simulink model "TwoLinkRobotOL"  (R2016b)
settings: Solver=VariableStepAuto  StartTime=0.0  StopTime=5  RelTol=1e-5
values from neighbouring files (symbols this model uses):
  alpha = RobotParam.alpha    [twoLinkInverseKinematics.m]    (also in twoLinkRobot_BuildLTVModel.m = 0.4425)
  beta = RobotParam.beta    [twoLinkInverseKinematics.m]    (also in twoLinkRobot_BuildLTVModel.m = 0.09)
  delta = RobotParam.delta    [twoLinkInverseKinematics.m]    (also in twoLinkRobot_BuildLTVModel.m = 0.105)
  eta0 = evalt(etabar,T0)    [twoLinkRobot_BuildLTVModel.m]
undefined symbols (not defined in the file): d, taubar
settings Model: Creator=pjseiler  LastModifiedBy=pjseiler

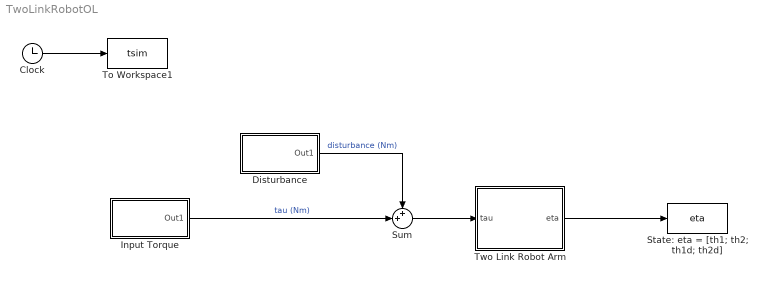
== system TwoLinkRobotOL ==
  Clock : Clock
  Disturbance : Subsystem  mask(Time-Varying Matrix){M=d, vec1D=on}
      mask prompts: M "Time-Varying Matrix"; vec1D "Interpret vector parameters as 1-D"
      mask help: Output the value of the specified time-varying matrix evaluated at the current simulation time. If the 'Time-Varying Matrix' parameter is M then the output at simulation time t is given by evalt(M,t). If M is a vector and the 'Interpret vector parameters as 1-D' is on, then the output is treated as a 1-D array. Otherwise the output is a matrix with the same dimensions as M.
      mask init:
      | if isequal(M.InterpolationMethod,'Spline') && ...
      |         isempty(M.SplineData)
      |     M = getSplineData(M);
      | end
      | fh = @(t) evalt(M,t);
      | szM = size(M);
      | if vec1D==1 && ndims(M)==2 && any(szM==1)
      |     dim = max(szM);
      | else
      |     dim = szM;
      | end
  Input Torque : Subsystem  mask(Time-Varying Matrix){M=taubar, vec1D=on}
      mask prompts: M "Time-Varying Matrix"; vec1D "Interpret vector parameters as 1-D"
      mask help: Output the value of the specified time-varying matrix evaluated at the current simulation time. If the 'Time-Varying Matrix' parameter is M then the output at simulation time t is given by evalt(M,t). If M is a vector and the 'Interpret vector parameters as 1-D' is on, then the output is treated as a 1-D array. Otherwise the output is a matrix with the same dimensions as M.
      mask init: same as TwoLinkRobotOL/Disturbance
  State: eta = [th1; th2; th1d; th2d] : ToWorkspace  VariableName=eta  SampleTime=-1
  Sum : Sum  Inputs=++|
  To Workspace1 : ToWorkspace  VariableName=tsim  SampleTime=-1
  Two Link Robot Arm : Subsystem
  wires:
  Disturbance/1(Out1) -> Sum/1  "disturbance (Nm)"
  Input Torque/1(Out1) -> Sum/2  "tau (Nm)"
  Clock/1 -> To Workspace1/1
  Sum/1 -> Two Link Robot Arm/1(tau)
  Two Link Robot Arm/1(eta) -> State: eta = [th1; th2; th1d; th2d]/1

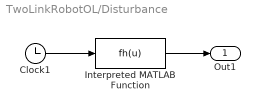
== system TwoLinkRobotOL/Disturbance ==
  Clock1 : Clock
  Interpreted MATLAB Function : MATLABFcn  MATLABFcn=fh(u)  OutputDimensions=dim  Output1D=off
  Out1 : Outport
  wires:
  Clock1/1 -> Interpreted MATLAB Function/1
  Interpreted MATLAB Function/1 -> Out1/1

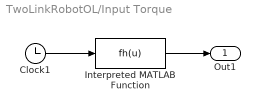
== system TwoLinkRobotOL/Input Torque ==
  Clock1 : Clock
  Interpreted MATLAB Function : MATLABFcn  MATLABFcn=fh(u)  OutputDimensions=dim  Output1D=off
  Out1 : Outport
  wires:
  Interpreted MATLAB Function/1 -> Out1/1
  Clock1/1 -> Interpreted MATLAB Function/1

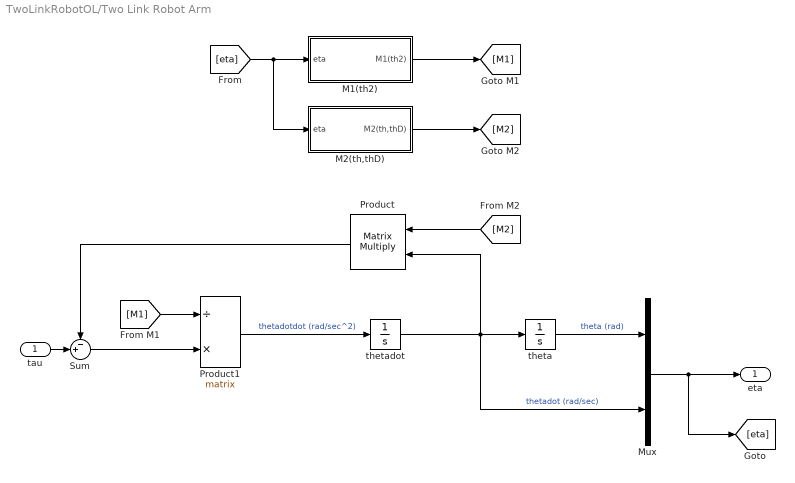
== system TwoLinkRobotOL/Two Link Robot Arm ==
  tau : Inport
  M1(th2) : Subsystem  TreatAsAtomicUnit=on
  M2(th,thD) : Subsystem  TreatAsAtomicUnit=on
  Mux : Mux  Inputs=2
  Product : Product  Inputs=**  Multiplication=Matrix(*)
  Product1 : Product  Inputs=/*  Multiplication=Matrix(*)
  Sum : Sum  Inputs=-+|
  theta : Integrator  InitialCondition=eta0(1:2)
  thetadot : Integrator  InitialCondition=eta0(3:4)
  eta : Outport
  wires:
  thetadot/1 -> Mux/2, Product/2, theta/1  "thetadot (rad/sec)"
  Sum/1 -> Product1/2
  Product/1 -> Sum/1
  [M1] -> Product1/1
  Product1/1 -> thetadot/1  "thetadotdot (rad/sec^2)"
  theta/1 -> Mux/1  "theta (rad)"
  M1(th2)/1(M1(th2)) -> [M1]
  [M2] -> Product/1
  M2(th,thD)/1(M2(th,thD)) -> [M2]
  [eta] -> M2(th,thD)/1(eta), M1(th2)/1(eta)
  Mux/1 -> [eta], eta/1
  tau/1 -> Sum/2

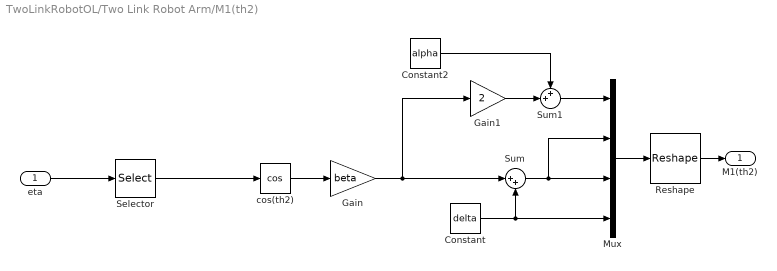
== system TwoLinkRobotOL/Two Link Robot Arm/M1(th2) ==
  eta : Inport
  Constant : Constant  Value=delta
  Constant2 : Constant  Value=alpha
  Gain : Gain  Gain=beta
  Gain1 : Gain  Gain=2
  Mux : Mux
  Reshape : Reshape  OutputDimensionality=Customize  OutputDimensions=[2 2]
  Selector : Selector  InputPortWidth=4  IndexOptions=Index vector (dialog)  Indices=2  OutputSizes=1
  Sum : Sum  Inputs=|++
  Sum1 : Sum  Inputs=++|
  cos(th2) : Trigonometry  Operator=cos
  M1(th2) : Outport
  wires:
  Reshape/1 -> M1(th2)/1
  Mux/1 -> Reshape/1
  Constant/1 -> Mux/4, Sum/2
  Sum/1 -> Mux/3, Mux/2
  cos(th2)/1 -> Gain/1
  Gain/1 -> Gain1/1, Sum/1
  Constant2/1 -> Sum1/1
  Sum1/1 -> Mux/1
  Gain1/1 -> Sum1/2
  eta/1 -> Selector/1
  Selector/1 -> cos(th2)/1

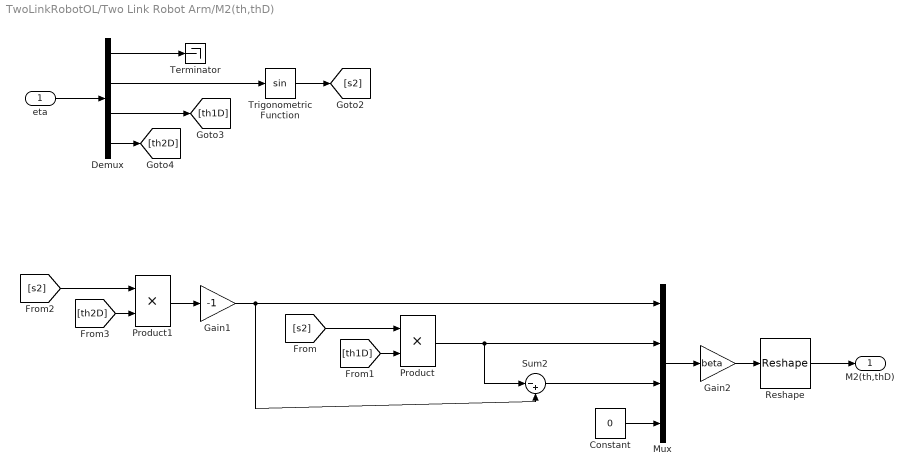
== system TwoLinkRobotOL/Two Link Robot Arm/M2(th,thD) ==
  eta : Inport
  Constant : Constant  Value=0
  Demux : Demux
  Gain1 : Gain  Gain=-1
  Gain2 : Gain  Gain=beta
  Mux : Mux
  Product : Product
  Product1 : Product
  Reshape : Reshape  OutputDimensionality=Customize  OutputDimensions=[2 2]
  Sum2 : Sum  Inputs=|-+
  Terminator : Terminator
  Trigonometric Function : Trigonometry
  M2(th,thD) : Outport
  wires:
  Constant/1 -> Mux/4
  Reshape/1 -> M2(th,thD)/1
  eta/1 -> Demux/1
  Demux/4 -> [th2D]
  Demux/1 -> Terminator/1
  Demux/2 -> Trigonometric Function/1
  Demux/3 -> [th1D]
  Trigonometric Function/1 -> [s2]
  [s2] -> Product/1
  [th1D] -> Product/2
  Product/1 -> Sum2/1, Mux/2
  Gain2/1 -> Reshape/1
  Mux/1 -> Gain2/1
  [th2D] -> Product1/2
  [s2] -> Product1/1
  Product1/1 -> Gain1/1
  Sum2/1 -> Mux/3
  Gain1/1 -> Sum2/2, Mux/1
